simulink model "BPSK"  (R2023b)
settings: Solver=ode45  StartTime=0.0  StopTime=20  MaxStep=0.01  MinStep=0.001  RelTol=1e-3  EnableMultiTasking=on
libraries: simulink x1
settings Model: Creator=SIMONA  LastModifiedBy=adiicmp_
settings SolverCC: AlgebraicLoopSolver=TrustRegion
settings DataIOCC: LimitDataPoints=on  SaveFormat=Array  ReturnWorkspaceOutputs=off
settings OptimizationCC: LifeSpan=inf
settings DebuggingCC: UnconnectedInputMsg=warning  UnconnectedOutputMsg=warning  UnconnectedLineMsg=warning  SFUnexpectedBacktrackingDiag=warning  SFNoUnconditionalDefaultTransitionDiag=warning  SFExecutionAtInitializationDiag=none  ArithmeticOperatorsInVariantConditions=warning
settings HardwareCC: ProdBitPerPointer=32  ProdBitPerSizeT=32  ProdBitPerPtrDiffT=32  ProdLargestAtomicFloat=None  ProdIntDivRoundTo=Undefined  ProdEndianess=Unspecified  ProdWordSize=32  ProdHWDeviceType=32-bit Generic
settings ModelReferenceCC: PropagateSignalLabelsOutOfModel=off
settings SFSimCC: SimUseLocalCustomCode=off  CustomCodeUndefinedFunction=UseInterfaceOnly
settings RTWCC: RTWUseLocalCustomCode=off
settings CodeAppCC: StateflowObjectComments=on
settings GRTTargetCC: TargetLangStandard=C89/C90 (ANSI)
settings ConfigComp: CovMetricSettings=dw  CovSaveCumulativeToWorkspaceVar=on  CovSaveSingleToWorkspaceVar=on  CovExternalEMLEnable=off

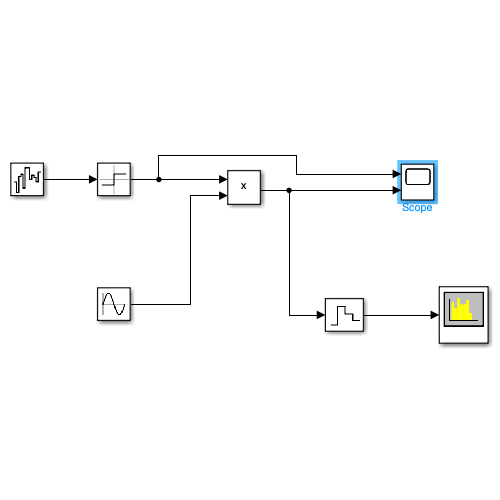
[thumbnail: Simulink's stored preview of the top-level diagram]
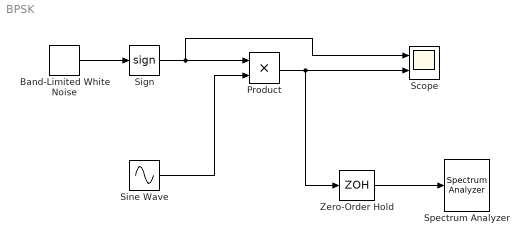
== system BPSK ==
  Band-Limited White Noise : simulink/Sources/Band-Limited White Noise  Cov=[0.1]  Ts=1  seed=[23341]
  Product : Product
  Scope : Scope  NumInputPorts=2
  Sign : Signum
  Sine Wave : Sin  Bias=4  Frequency=2*pi*10  SampleTime=0
  Spectrum Analyzer : SpectrumAnalyzer  WindowPosition=[320.000000,200.000000,800.000000,500.000000,]  ScopeFrameLocation=window  SpectrumType=Power density  Method=Welch  SampleRate=100  AxesScaling=Manual  Span=100  StartFrequency=-50  StopFrequency=50  AveragingMethod=Running  SpectrumUnits=dBm/Hz  YLabel=dBm / Hz  YLimits=[-43.928529500137167,34.152532005572709]  ShowGrid=off  SelectedToolstripTab=spectrumAnalyzerToolstrip.spectrumTab  DefaultConfigurationName=spbscopes.SpectrumAnalyzerBlockCfg
  Zero-Order Hold : ZeroOrderHold  SampleTime=0.01
  wires:
  Band-Limited White Noise/1 -> Sign/1
  Sign/1 -> Scope/1, Product/1
  Sine Wave/1 -> Product/2
  Product/1 -> Zero-Order Hold/1, Scope/2
  Zero-Order Hold/1 -> Spectrum Analyzer/1
